simulink model "double_integrator_plant"  (R2021b)
settings: Solver=VariableStepAuto  StartTime=0.0  StopTime=10.0  RelTol=1e-3
settings Model: Creator=AaronLey  LastModifiedBy=AaronLey

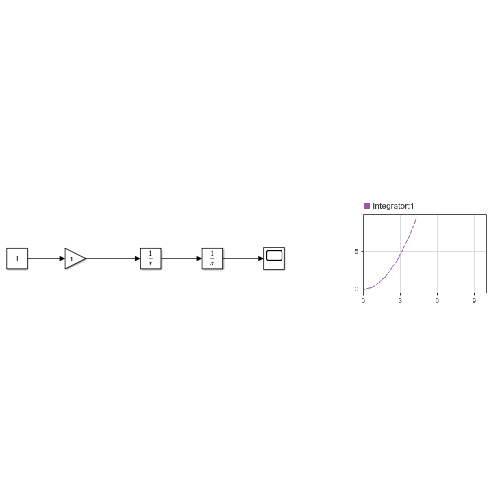
[thumbnail: Simulink's stored preview of the top-level diagram]
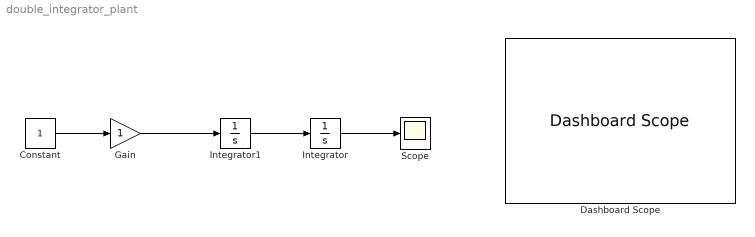
== system double_integrator_plant ==
  Constant : Constant
  Dashboard Scope : DashboardScope
  Gain : Gain
  Integrator : Integrator
  Integrator1 : Integrator
  Scope : Scope
  wires:
  Integrator1/1 -> Integrator/1
  Constant/1 -> Gain/1
  Gain/1 -> Integrator1/1
  Integrator/1 -> Scope/1
